simulink model "pend1"  (R2021b)
settings: Solver=VariableStepAuto  StartTime=0.0  StopTime=100.0  RelTol=1e-3
undefined symbols (not defined in the file): g, l, M, m
settings Model: Creator=vladimirberman  LastModifiedBy=vladimirberman

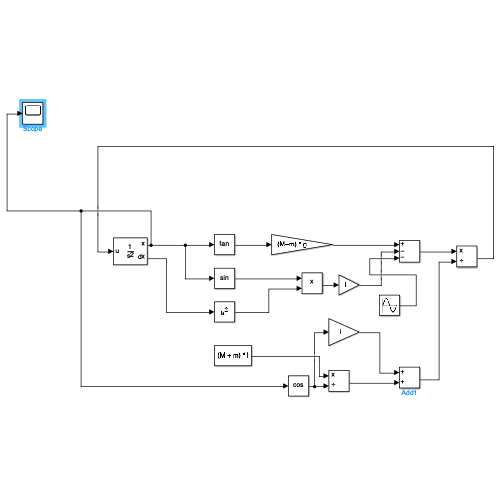
[thumbnail: Simulink's stored preview of the top-level diagram]
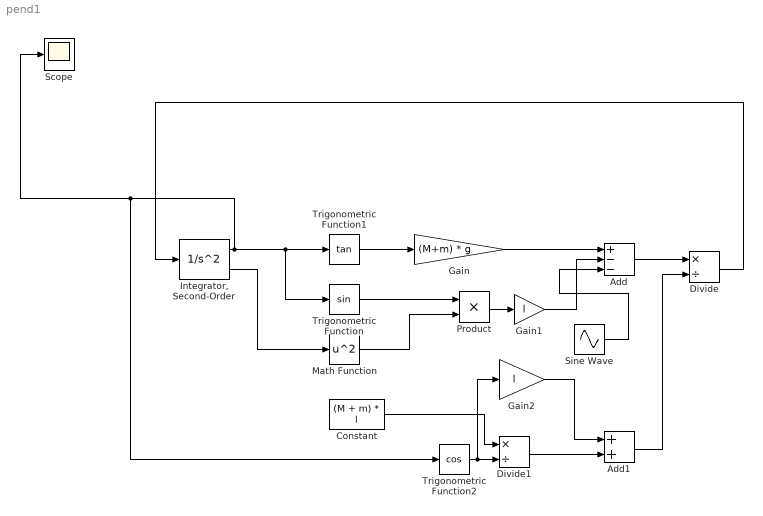
== system pend1 ==
  Add : Sum  Inputs=+--
  Add1 : Sum
  Constant : Constant  Value=(M + m) * l
  Divide : Product  Inputs=*/
  Divide1 : Product  Inputs=*/
  Gain : Gain  Gain=(M+m) * g
  Gain1 : Gain  Gain=l
  Gain2 : Gain  Gain=l
  "Integrator, Second-Order" : SecondOrderIntegrator  ICX=0.01
  Math Function : Math  Operator=square  SaturateOnIntegerOverflow=on
  Product : Product
  Scope : Scope
  Sine Wave : Sin  Amplitude=0.3  SampleTime=0
  Trigonometric Function : Trigonometry
  Trigonometric Function1 : Trigonometry  Operator=tan
  Trigonometric Function2 : Trigonometry  Operator=cos
  wires:
  Trigonometric Function1/1 -> Gain/1
  Gain/1 -> Add/1
  Trigonometric Function/1 -> Product/1
  Product/1 -> Gain1/1
  Gain1/1 -> Add/2
  Math Function/1 -> Product/2
  "Integrator, Second-Order"/2 -> Math Function/1
  Add/1 -> Divide/1
  Constant/1 -> Divide1/1
  Trigonometric Function2/1 -> Divide1/2, Gain2/1
  "Integrator, Second-Order"/1 -> Trigonometric Function/1, Trigonometric Function1/1, Scope/1, Trigonometric Function2/1
  Divide1/1 -> Add1/2
  Gain2/1 -> Add1/1
  Add1/1 -> Divide/2
  Divide/1 -> "Integrator, Second-Order"/1
  Sine Wave/1 -> Add/3
